simulink model "PFmsr_TDPA_TD"  (R2021b)
settings: Solver=FixedStepAuto  StartTime=0.0  StopTime=20  FixedStep=0.001  RelTol=1e-3
settings Model: Creator=lucao  LastModifiedBy=lucao

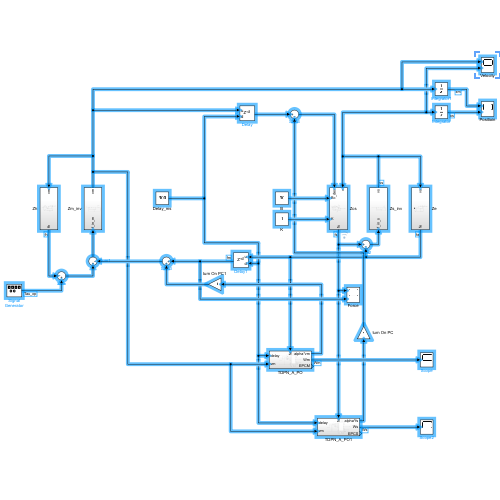
[thumbnail: Simulink's stored preview of the top-level diagram]
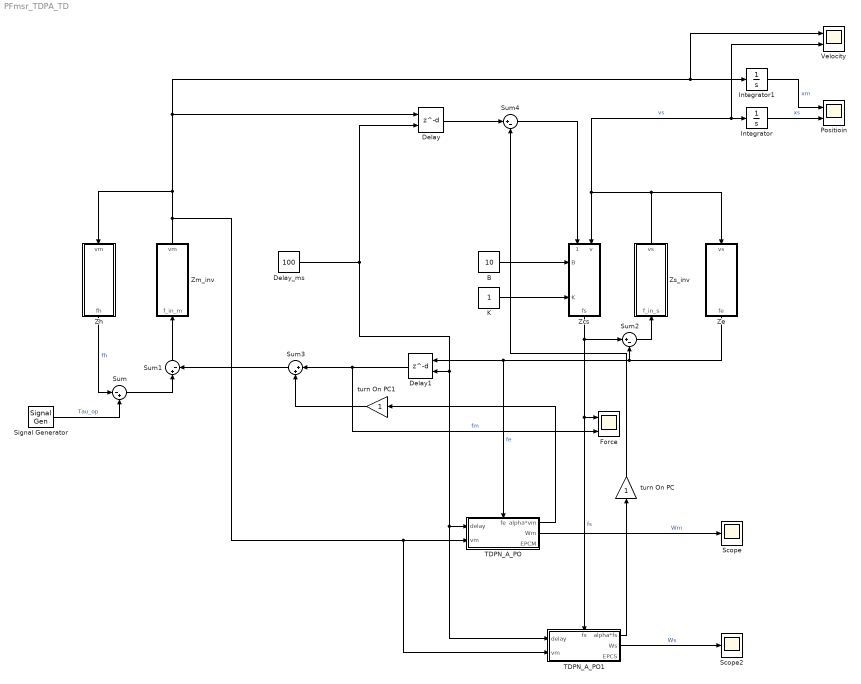
== system PFmsr_TDPA_TD ==
  B : Constant  Value=10
  Delay : Delay  DelayLengthSource=Input port  DelayLength=100  DelayLengthUpperLimit=10000
      settings: InputPortMap=u0,p1
  Delay1 : Delay  DelayLengthSource=Input port  DelayLength=100  DelayLengthUpperLimit=10000
      settings: InputPortMap=u0,p1
  Delay_ms : Constant  Value=100
  Force : Scope  NumInputPorts=2
  Integrator : Integrator
  Integrator1 : Integrator
  K : Constant
  Positioin : Scope  NumInputPorts=2
  Scope : Scope
  Scope2 : Scope
  Signal Generator : SignalGenerator  Amplitude=10  Frequency=0.25
  Sum : Sum  Inputs=|-+
  Sum1 : Sum  Inputs=|+-
  Sum2 : Sum  Inputs=|+-
  Sum3 : Sum  Inputs=|++
  Sum4 : Sum  Inputs=|+-
  TDPN_A_PO : Subsystem
      settings: PortSchema="{\"entries\":[{\"content\":{\"sides\":[{\"content\":{\"connectorIds\":[\"In1\",\"In2\"]},\"type\":\"ConnectorPlacement.EquallySpacedRectSide\",\"uuid\":\"f0b554bf-d147-4333-ac0a-083af6ae8427\"},{\"content\":{\"connectorIds\":[\"Out1\",\"Out2\",\"Out3\"],\"side\":\"RIGHT\"},\"type\":\"ConnectorPlacement.EquallySpacedRectSide\",\"uuid\":\"78fd55c3-bf7c-4f3c-baf7-a1fc5c1f44e2\"},{\"content\":{\"connectorIds\":[\"In3\"],\"side\":\"TOP\"},\"type\":\"ConnectorPlacement.EquallySpacedRectSide\",\"uuid\":\"342b47c6-54e7-4705-ba9a-6aca32ab5776\"}]},\"type\":\"ConnectorPlacement.EquallySpacedConnector\",\"uuid\":\"921b42e7-f3a1-4f05-a13a-b8fe1fb9d8b5\"}],\"packageUris\":[\"http://schema.mathworks.com/mf0/Connector/R2020b\"],\"version\":\"1.0\"}"
  TDPN_A_PO1 : Subsystem
      settings: PortSchema="{\"entries\":[{\"content\":{\"sides\":[{\"content\":{\"connectorIds\":[\"In1\",\"In2\"]},\"type\":\"ConnectorPlacement.EquallySpacedRectSide\",\"uuid\":\"f0b554bf-d147-4333-ac0a-083af6ae8427\"},{\"content\":{\"connectorIds\":[\"Out1\",\"Out2\",\"Out3\"],\"side\":\"RIGHT\"},\"type\":\"ConnectorPlacement.EquallySpacedRectSide\",\"uuid\":\"78fd55c3-bf7c-4f3c-baf7-a1fc5c1f44e2\"},{\"content\":{\"connectorIds\":[\"In3\"],\"side\":\"TOP\"},\"type\":\"ConnectorPlacement.EquallySpacedRectSide\",\"uuid\":\"342b47c6-54e7-4705-ba9a-6aca32ab5776\"}]},\"type\":\"ConnectorPlacement.EquallySpacedConnector\",\"uuid\":\"921b42e7-f3a1-4f05-a13a-b8fe1fb9d8b5\"}],\"packageUris\":[\"http://schema.mathworks.com/mf0/Connector/R2020b\"],\"version\":\"1.0\"}"
  Velocity : Scope  NumInputPorts=2
  Zcs : Subsystem
      settings: PortSchema="{\"entries\":[{\"content\":{\"sides\":[{\"content\":{\"connectorIds\":[\"In1\",\"In2\"]},\"type\":\"ConnectorPlacement.EquallySpacedRectSide\",\"uuid\":\"c32e4091-a441-4f3b-b0b8-cebe01d42adf\"},{\"content\":{\"connectorIds\":[\"Out1\"],\"side\":\"RIGHT\"},\"type\":\"ConnectorPlacement.EquallySpacedRectSide\",\"uuid\":\"ccadc46e-4cdd-4994-a822-3ba84443801c\"},{\"content\":{\"connectorIds\":[\"In3\",\"In4\"],\"side\":\"TOP\"},\"type\":\"ConnectorPlacement.EquallySpacedRectSide\",\"uuid\":\"020656f3-557f-4da7-a585-94cb368715db\"}]},\"type\":\"ConnectorPlacement.EquallySpacedConnector\",\"uuid\":\"4a9455fd-3018-4498-b276-9155c948801a\"}],\"packageUris\":[\"http://schema.mathworks.com/mf0/Connector/R2020b\"],\"version\":\"1.0\"}"
  Ze : Subsystem
  Zh : Subsystem
  Zm_inv : Subsystem
  Zs_inv : Subsystem
  turn On PC : Gain
  turn On PC1 : Gain
  wires:
  Zs_inv/1(vs) -> Zcs/2(v), Velocity/2, Integrator/1, Ze/1(vs)  "vs"
  Sum1/1 -> Zm_inv/1(f_in_m)
  Zcs/1(fs) -> TDPN_A_PO1/3(fs), Force/1, Sum2/1  "fs"
  Sum2/1 -> Zs_inv/1(f_in_s)
  Ze/1(fe) -> Delay1/1, TDPN_A_PO/3(fe), Sum2/2  "fe"
  Integrator1/1 -> Positioin/1  "xm"
  Integrator/1 -> Positioin/2  "xs"
  Zm_inv/1(vm) -> TDPN_A_PO1/2(vm), TDPN_A_PO/2(vm), Delay/1, Velocity/1, Integrator1/1, Zh/1(vm)
  Zh/1(fh) -> Sum/1  "fh"
  Signal Generator/1 -> Sum/2  "Tau_op"
  Sum/1 -> Sum1/1
  B/1 -> Zcs/3(B)
  K/1 -> Zcs/4(K)
  Delay1/1 -> Sum3/1, Force/2  "fm"
  Delay_ms/1 -> TDPN_A_PO1/1(delay), TDPN_A_PO/1(delay), Delay1/2, Delay/2
  TDPN_A_PO/1(alpha*vm) -> turn On PC1/1
  Sum3/1 -> Sum1/2
  TDPN_A_PO/2(Wm) -> Scope/1  "Wm"
  Delay/1 -> Sum4/1
  Sum4/1 -> Zcs/1(v_des)
  TDPN_A_PO1/1(alpha*fs) -> turn On PC/1
  turn On PC/1 -> Sum4/2
  turn On PC1/1 -> Sum3/2
  TDPN_A_PO1/2(Ws) -> Scope2/1  "Ws"

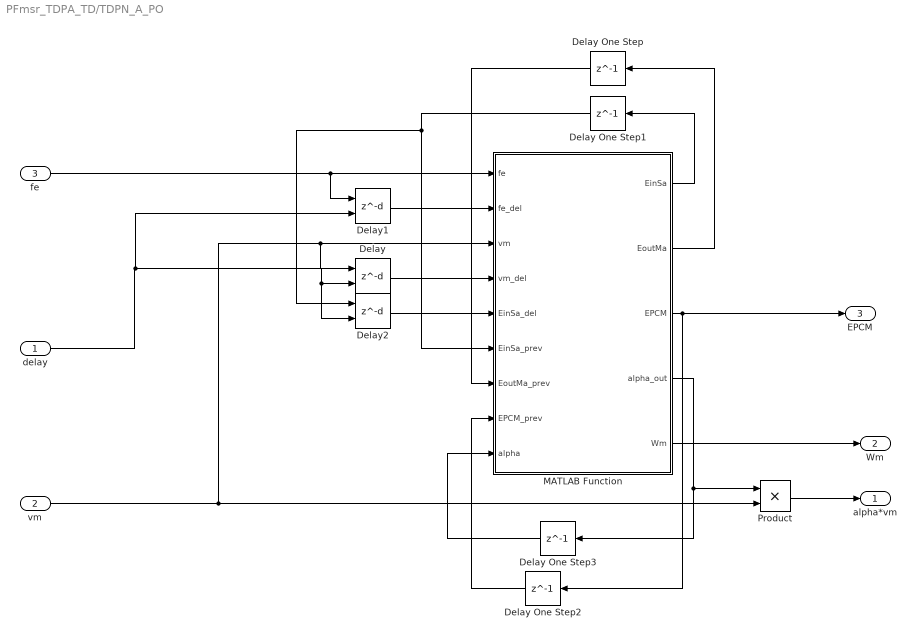
== system PFmsr_TDPA_TD/TDPN_A_PO ==
  delay : Inport
  vm : Inport  Port=2
  fe : Inport  Port=3
  Delay : Delay  DelayLengthSource=Input port
      settings: InputPortMap=u0,p1
  Delay One Step{,1..3} (4 alike) : Delay  DelayLength=1
  Delay1 : Delay  DelayLengthSource=Input port
      settings: InputPortMap=u0,p1
  Delay2 : Delay  DelayLengthSource=Input port
      settings: InputPortMap=u0,p1
  MATLAB Function : MATLAB Function  TreatAsAtomicUnit=on
  Product : Product
  alpha*vm : Outport
  Wm : Outport  Port=2
  EPCM : Outport  Port=3
  wires:
  Product/1 -> alpha*vm/1
  MATLAB Function/4(alpha_out) -> Product/1, Delay One Step3/1
  vm/1 -> Product/2, Delay/1, MATLAB Function/3(vm)
  delay/1 -> Delay1/2, Delay2/2, Delay/2
  Delay/1 -> MATLAB Function/4(vm_del)
  fe/1 -> Delay1/1, MATLAB Function/1(fe)
  Delay1/1 -> MATLAB Function/2(fe_del)
  MATLAB Function/1(EinSa) -> Delay One Step1/1
  Delay2/1 -> MATLAB Function/5(EinSa_del)
  MATLAB Function/2(EoutMa) -> Delay One Step/1
  MATLAB Function/3(EPCM) -> Delay One Step2/1, EPCM/1
  Delay One Step/1 -> MATLAB Function/7(EoutMa_prev)
  Delay One Step1/1 -> MATLAB Function/6(EinSa_prev), Delay2/1
  Delay One Step2/1 -> MATLAB Function/8(EPCM_prev)
  Delay One Step3/1 -> MATLAB Function/9(alpha)
  MATLAB Function/5(Wm) -> Wm/1

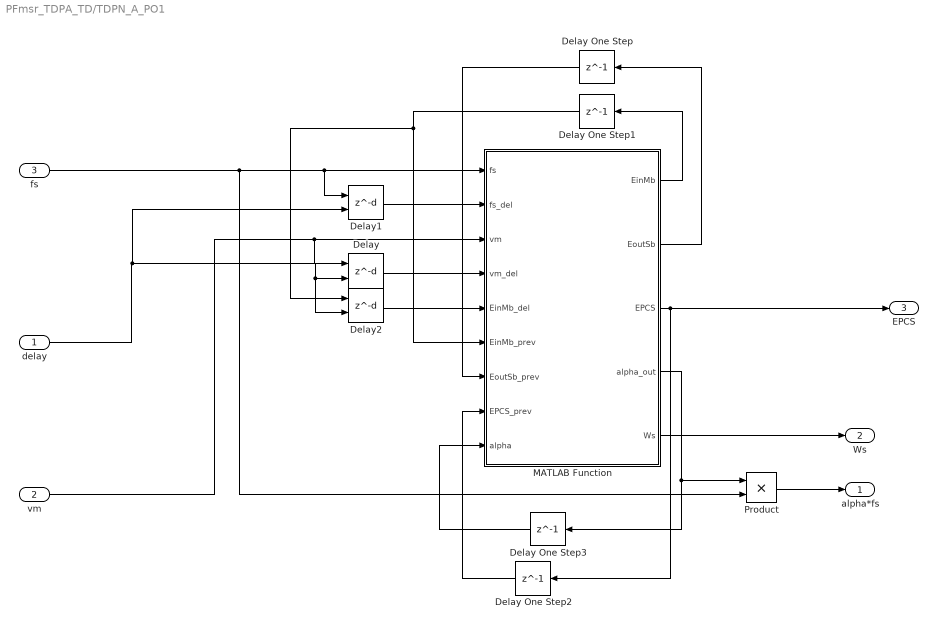
== system PFmsr_TDPA_TD/TDPN_A_PO1 ==
  delay : Inport
  vm : Inport  Port=2
  fs : Inport  Port=3
  Delay : Delay  DelayLengthSource=Input port
      settings: InputPortMap=u0,p1
  Delay One Step{,1..3} (4 alike) : Delay  DelayLength=1
  Delay1 : Delay  DelayLengthSource=Input port
      settings: InputPortMap=u0,p1
  Delay2 : Delay  DelayLengthSource=Input port
      settings: InputPortMap=u0,p1
  MATLAB Function : MATLAB Function  TreatAsAtomicUnit=on
  Product : Product
  alpha*fs : Outport
  Ws : Outport  Port=2
  EPCS : Outport  Port=3
  wires:
  Product/1 -> alpha*fs/1
  MATLAB Function/4(alpha_out) -> Product/1, Delay One Step3/1
  vm/1 -> Delay/1, MATLAB Function/3(vm)
  delay/1 -> Delay1/2, Delay2/2, Delay/2
  Delay/1 -> MATLAB Function/4(vm_del)
  fs/1 -> Product/2, Delay1/1, MATLAB Function/1(fs)
  Delay1/1 -> MATLAB Function/2(fs_del)
  MATLAB Function/1(EinMb) -> Delay One Step1/1
  Delay2/1 -> MATLAB Function/5(EinMb_del)
  MATLAB Function/2(EoutSb) -> Delay One Step/1
  MATLAB Function/3(EPCS) -> Delay One Step2/1, EPCS/1
  Delay One Step/1 -> MATLAB Function/7(EoutSb_prev)
  Delay One Step1/1 -> MATLAB Function/6(EinMb_prev), Delay2/1
  Delay One Step2/1 -> MATLAB Function/8(EPCS_prev)
  Delay One Step3/1 -> MATLAB Function/9(alpha)
  MATLAB Function/5(Ws) -> Ws/1

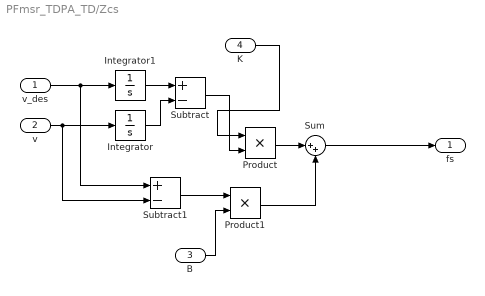
== system PFmsr_TDPA_TD/Zcs ==
  v_des : Inport
  v : Inport  Port=2
  B : Inport  Port=3
  K : Inport  Port=4
  Integrator : Integrator
  Integrator1 : Integrator
  Product : Product
  Product1 : Product
  Subtract : Sum  Inputs=+-
  Subtract1 : Sum  Inputs=+-
  Sum : Sum  Inputs=|++
  fs : Outport
  wires:
  v_des/1 -> Integrator1/1, Subtract1/1
  v/1 -> Subtract1/2, Integrator/1
  Subtract/1 -> Product/2
  Subtract1/1 -> Product1/1
  Product/1 -> Sum/1
  Product1/1 -> Sum/2
  Sum/1 -> fs/1
  Integrator/1 -> Subtract/2
  Integrator1/1 -> Subtract/1
  K/1 -> Product/1
  B/1 -> Product1/2

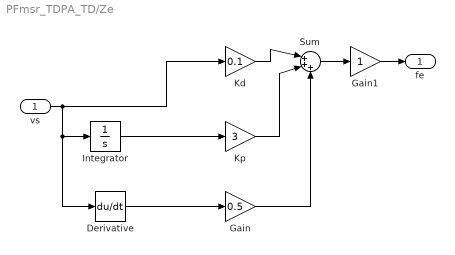
== system PFmsr_TDPA_TD/Ze ==
  vs : Inport
  Derivative : Derivative
  Gain : Gain  Gain=0.5
  Gain1 : Gain
  Integrator : Integrator
  Kd : Gain  Gain=0.1
  Kp : Gain  Gain=3
  Sum : Sum  Inputs=|+++
  fe : Outport
  wires:
  vs/1 -> Derivative/1, Integrator/1, Kd/1
  Kp/1 -> Sum/2
  Kd/1 -> Sum/1
  Sum/1 -> Gain1/1
  Gain/1 -> Sum/3
  Gain1/1 -> fe/1
  Integrator/1 -> Kp/1
  Derivative/1 -> Gain/1

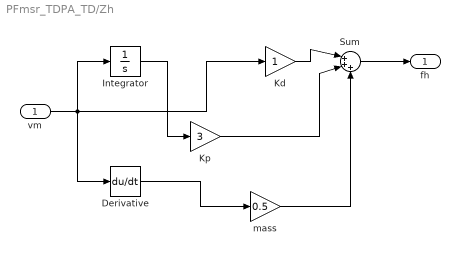
== system PFmsr_TDPA_TD/Zh ==
  vm : Inport
  Derivative : Derivative
  Integrator : Integrator
  Kd : Gain
  Kp : Gain  Gain=3
  Sum : Sum  Inputs=|+++
  mass : Gain  Gain=0.5
  fh : Outport
  wires:
  Kp/1 -> Sum/2
  Kd/1 -> Sum/1
  Sum/1 -> fh/1
  Integrator/1 -> Kp/1
  Derivative/1 -> mass/1
  mass/1 -> Sum/3
  vm/1 -> Derivative/1, Integrator/1, Kd/1

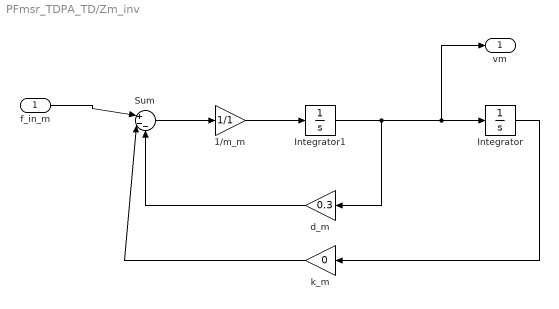
== system PFmsr_TDPA_TD/Zm_inv ==
  f_in_m : Inport
  1/m_m : Gain  Gain=1/1
  Integrator : Integrator
  Integrator1 : Integrator
  Sum : Sum  Inputs=|+--
  d_m : Gain  Gain=0.3
  k_m : Gain  Gain=0
  vm : Outport
  wires:
  Integrator/1 -> k_m/1
  Integrator1/1 -> d_m/1, vm/1, Integrator/1
  f_in_m/1 -> Sum/1
  d_m/1 -> Sum/3
  k_m/1 -> Sum/2
  Sum/1 -> 1/m_m/1
  1/m_m/1 -> Integrator1/1

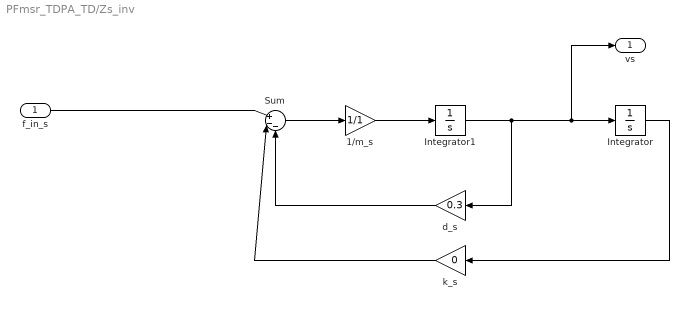
== system PFmsr_TDPA_TD/Zs_inv ==
  f_in_s : Inport
  1/m_s : Gain  Gain=1/1
  Integrator : Integrator
  Integrator1 : Integrator
  Sum : Sum  Inputs=|+--
  d_s : Gain  Gain=0.3
  k_s : Gain  Gain=0
  vs : Outport
  wires:
  Integrator/1 -> k_s/1
  Integrator1/1 -> d_s/1, vs/1, Integrator/1
  f_in_s/1 -> Sum/1
  d_s/1 -> Sum/3
  k_s/1 -> Sum/2
  Sum/1 -> 1/m_s/1
  1/m_s/1 -> Integrator1/1

== matlab function PFmsr_TDPA_TD/TDPN_A_PO1/MATLAB Function ==
  data: fs input; EinMb output; fs_del input; vm input; vm_del input; EinMb_del input; EinMb_prev input; EoutSb_prev input; EPCS_prev input; alpha input; EoutSb output; EPCS output; alpha_out output; Ws output
function [EinMb, EoutSb, EPCS, alpha_out, Ws] = fcn(fs,fs_del, vm, vm_del, EinMb_del, EinMb_prev, EoutSb_prev,EPCS_prev, alpha)

    if (fs_del*vm>0)
        PinMb = fs_del*vm;
    else
        PinMb = 0;
    end
    if (-fs*vm_del<0)
        PoutSb = fs*vm_del;
    else
        PoutSb = 0;
    end
    EinMb = EinMb_prev + 0.001*PinMb;
    EoutSb = EoutSb_prev + 0.001*PoutSb;

    EPCS = EPCS_prev + 0.001*fs^2*alpha;

    Ws = EinMb_del - EoutSb + EPCS;

    if (Ws>0)
        alpha_out = 0;
    else
        if (fs~=0)
            alpha_out = -Ws/(0.001*fs^2);
        else
            alpha_out = 0;
        end
    end

== matlab function PFmsr_TDPA_TD/TDPN_A_PO/MATLAB Function ==
  data: fe input; EinSa output; fe_del input; vm input; vm_del input; EinSa_del input; EinSa_prev input; EoutMa_prev input; EPCM_prev input; alpha input; EoutMa output; EPCM output; alpha_out output; Wm output
function [EinSa, EoutMa, EPCM, alpha_out, Wm] = fcn(fe,fe_del, vm, vm_del, EinSa_del, EinSa_prev, EoutMa_prev,EPCM_prev, alpha)

    if (-fe*vm_del>0)
        PinSa = -fe*vm_del;
    else
        PinSa = 0;
    end
    if (fe_del*vm<0)
        PoutMa = -fe_del*vm;
    else
        PoutMa = 0;
    end
    EinSa = EinSa_prev + 0.001*PinSa;
    EoutMa = EoutMa_prev + 0.001*PoutMa;

    EPCM = EPCM_prev + 0.001*vm^2*alpha;

    Wm = EinSa_del - EoutMa + EPCM;

    if (Wm>0)
        alpha_out = 0;
    else
        if (vm~=0)
            alpha_out = -Wm/(0.001*vm^2);
        else
            alpha_out = 0;
        end
    end
